simulink model "mpc_model_dual_module_allfreq"  (R2019a)
settings: Solver=FixedStepAuto  StartTime=0.0  StopTime=Tfinal  RelTol=1e-3
values from neighbouring files (symbols this model uses):
  A = [-0.0285 -0.0014; -0.0371 -0.1476]    [model.m]
  DCLINK_Cap = 1000e-12    (= 1e-09)    [mpc_model_parameters.m]    (also in mpc_model_parameters_dual_module.m = 0.001)
  FluxPM = MeanInducedVoltagePeak/(2*pi*100)    [mpc_model_parameters.m]    (also in mpc_model_parameters_dual_module.m)
  Inertia = 1e-2    (= 0.01)    [mpc_model_parameters.m]    (also in mpc_model_parameters_dual_module.m)
  iqrated = Trated/(1.5*PolePairs*FluxPM)    [mpc_model_parameters.m]    (also in mpc_model_parameters_dual_module.m)
  Ki = 8    [mpc_model_parameters_dual_module.m]
  Kp = 0.8    [mpc_model_parameters_dual_module.m]
  Ls = 3.5e-3    (= 0.0035)    [MPC_id_iq.m]    (also in mpc_model_parameters.m = 0.00351; mpc_model_parameters_dual_module.m = 0.00343)
  M1_FaultTime = 0.25    [mpc_model_parameters_dual_module.m]
  M2_FaultTime = 20    [mpc_model_parameters_dual_module.m]
  MeanLd = (1/12)*(Module1Phase_A_Ld+Module1Phase_B_Ld+Module1Phase_C_Ld+     Module2Phase_A_Ld+Module2Phase_B_Ld+Module2Phase_C_Ld+     Module3Phase_A_Ld+Module3Phase_B_Ld+Module3Phase_C_Ld+     Module4Phase_A_Ld+Module4Phase_B_Ld+Module4Phase_C_Ld)    [mpc_model_parameters.m]    (also in mpc_model_parameters_dual_module.m)
  MeanLq = (1/12)*(Module1Phase_A_Lq+Module1Phase_B_Lq+Module1Phase_C_Lq+     Module2Phase_A_Lq+Module2Phase_B_Lq+Module2Phase_C_Lq+     Module3Phase_A_Lq+Module3Phase_B_Lq+Module3Phase_C_Lq+     Module4Phase_A_Lq+Module4Phase_B_Lq+Module4Phase_C_Lq)    [mpc_model_parameters.m]    (also in mpc_model_parameters_dual_module.m)
  PI_Frequency = 5000    [mpc_model_parameters_dual_module.m]
  PI_Sat = iqrated*2    [mpc_model_parameters_dual_module.m]
  PI_Ts = 1/PI_Frequency    (= 0.0002)    [mpc_model_parameters_dual_module.m]
  PolePairs = 10    [mpc_model_parameters.m]    (also in mpc_model_parameters_dual_module.m)
  RefModeSelection = 1    [mpc_model_parameters_dual_module.m]
  Rin = 1e-3    (= 0.001)    [mpc_model_parameters.m]    (also in mpc_model_parameters_dual_module.m)
  Rs = 0.531    [Loss_Distribution.m]    (also in MPC_id_iq.m; mpc_model_parameters.m = 0.321; mpc_model_parameters_dual_module.m = 0.539)
  Sampling_time = 1e-6    (= 1e-06)    [mpc_model_parameters.m]    (also in mpc_model_parameters_dual_module.m)
  SpeedRef1 = 50    [mpc_model_parameters.m]    (also in mpc_model_parameters_dual_module.m = 35)
  SpeedRef2 = 100    [mpc_model_parameters.m]    (also in mpc_model_parameters_dual_module.m = 35)
  SpeedRefUpdateTime = 0.25    [mpc_model_parameters.m]    (also in mpc_model_parameters_dual_module.m = 1.75)
  Tload1 = 5    [mpc_model_parameters.m]    (also in mpc_model_parameters_dual_module.m = 30)
  Tload2 = 10    [mpc_model_parameters.m]    (also in mpc_model_parameters_dual_module.m = 63.6619772368)
  TloadUpdateTime = 0.5    [mpc_model_parameters.m]    (also in mpc_model_parameters_dual_module.m)
  Vdc = 50    [mpc_model_parameters.m]    (also in mpc_model_parameters_dual_module.m = 40)
  Vin = Vdc + Rin*(Pout/Vdc)    (= 50.04)    [mpc_model_parameters.m]    (also in mpc_model_parameters_dual_module.m = 40.05)
  ViscousFriction = 1e-3    (= 0.001)    [mpc_model_parameters.m]    (also in mpc_model_parameters_dual_module.m)
undefined symbols (not defined in the file or in its folder): DiscIntNeverNeededParam
libraries: powerlib x27, dspsigops x21, dspswit3 x19, powerlib_meascontrol x10, fl_lib x5, simulink x4, nesl_utility x3, sdl_lib x1
(part 3 of 3)

== matlab function mpc_model_dual_module_allfreq/MATLAB Function1 ==
  data: pulse input; inputwave input; outputwave output
function outputwave  = fcn(pulse, inputwave)

persistent state

if isempty(state)
state = 0;
end

if(pulse==1)
    state = state +1;
end

if(mod(state,2)==1)
    outputwave = inputwave;
    return;
end
if(mod(state,2)==0)
    outputwave = 1-inputwave;
    return;
end

outputwave = 5;

== matlab function mpc_model_dual_module_allfreq/MATLAB Function2 ==
  data: pulse input; inputwave input; outputwave output
function outputwave  = fcn(pulse, inputwave)

persistent state

if isempty(state)
state = 0;
end

if(pulse==1)
    state = state +1;
end

if(mod(state,2)==1)
    outputwave = inputwave;
    return;
end
if(mod(state,2)==0)
    outputwave = 1-inputwave;
    return;
end

outputwave = 5;

== matlab function mpc_model_dual_module_allfreq/module 1 abc to dq1 ==
  data: ids output; iqs output; ias input; ibs input; ics input; ref_frame_position input; i0 output
function [ids,iqs,i0 ]  = fcn(ias,ibs,ics,ref_frame_position)





ids = 2/3*(ias*sin(ref_frame_position)+ibs*sin(ref_frame_position-2*pi/3)+ics*sin(ref_frame_position+2*pi/3));
iqs =  2/3*(ias*cos(ref_frame_position)+ibs*cos(ref_frame_position-2*pi/3)+ics*cos(ref_frame_position+2*pi/3));
i0 = 2/3*1/2*(ias+ibs+ics);
% iqs = (vqs-fluxlinkage_qs_derivative-ref_frame_velocity*fluxlinkage_ds)/rs;
% ids = (vds-fluxlinkage_ds_derivative+ref_frame_velocity*fluxlinkage_qs)/rs;

== matlab function mpc_model_dual_module_allfreq/MATLAB Function4 ==
  data: M1_ia input; M1_loss output; M1_ib input; M1_ic input; M2_ia input; M2_ib input; M2_ic input; M2_loss output; Total_loss output; Rs input
function [M1_loss,M2_loss,Total_loss] = fcn(M1_ia, M1_ib, M1_ic, M2_ia, M2_ib, M2_ic, Rs)



M1_loss = Rs*(M1_ia^2+M1_ib^2+M1_ic^2);
M2_loss = Rs*(M2_ia^2+M2_ib^2+M2_ic^2);
Total_loss = M1_loss+M2_loss;

== matlab function mpc_model_dual_module_allfreq/MATLAB Function5 ==
  data: M1_ids input; M1_magnetic_loss output; M1_iqs input; M2_ids input; M2_iqs input; FluxPM input; Ls input; ElectricalSpeed input; M2_magnetic_loss output; Total_loss output
function [M1_magnetic_loss,M2_magnetic_loss,Total_loss] = fcn(M1_ids,M1_iqs,M2_ids,M2_iqs,FluxPM,Ls,ElectricalSpeed)

cfe = 1.55;
lambda = 1.55;
M1_d_axis_flux = Ls*M1_ids+FluxPM;
M1_q_axis_flux = Ls*M1_iqs;
M2_d_axis_flux = Ls*M2_ids+FluxPM;
M2_q_axis_flux = Ls*M2_iqs;

M1_magnetic_loss = cfe*power(abs(ElectricalSpeed),lambda)*(M1_d_axis_flux^2+M1_q_axis_flux^2);
M2_magnetic_loss = cfe*power(abs(ElectricalSpeed),lambda)*(M2_d_axis_flux^2+M2_q_axis_flux^2);

% M1_loss = Rs*(M1_ia^2+M1_ib^2+M1_ic^2);
% M2_loss = Rs*(M2_ia^2+M2_ib^2+M2_ic^2);
Total_loss = M1_magnetic_loss+M2_magnetic_loss;

== matlab function mpc_model_dual_module_allfreq/MATLAB Function6 ==
  data: pulse input; inputwave input; outputwave output
function outputwave  = fcn(pulse, inputwave)

persistent state

if isempty(state)
state = 0;
end

if(pulse==1)
    state = state +1;
end

if(mod(state,2)==1)
    outputwave = inputwave;
    return;
end
if(mod(state,2)==0)
    outputwave = 1-inputwave;
    return;
end

outputwave = 5;

== matlab function mpc_model_dual_module_allfreq/MATLAB Function7 ==
  data: M1_Iq_opt_cost input; M1_iqref output; M1_Id_opt_cost input; M2_Iq_opt_cost input; M2_Id_opt_cost input; M1_Iq_opt_proportional input; M1_Id_opt_proportional input; M2_Iq_opt_proportional input; M2_Id_opt_proportional input; M1_Iq_opt_equal input; M1_Id_opt_equal input; M2_Iq_opt_equal input; M2_Id_opt_equal input; M1_idref output; M2_iqref output; M2_idref output; selection input
function [M1_iqref, M1_idref, M2_iqref, M2_idref] = fcn(M1_Iq_opt_cost,M1_Id_opt_cost,M2_Iq_opt_cost,M2_Id_opt_cost...
    ,M1_Iq_opt_proportional,M1_Id_opt_proportional,M2_Iq_opt_proportional,M2_Id_opt_proportional,...
    M1_Iq_opt_equal,M1_Id_opt_equal,M2_Iq_opt_equal,M2_Id_opt_equal,selection)


if(selection==1)
    M1_iqref = M1_Iq_opt_cost;
    M1_idref = M1_Id_opt_cost;
    M2_iqref = M2_Iq_opt_cost;
    M2_idref = M2_Id_opt_cost;
    return
end


if(selection==2)
    M1_iqref = M1_Iq_opt_proportional;
    M1_idref = M1_Id_opt_proportional;
    M2_iqref = M2_Iq_opt_proportional;
    M2_idref = M2_Id_opt_proportional;
    return
end



if(selection==3)
    M1_iqref = M1_Iq_opt_equal;
    M1_idref = M1_Id_opt_equal;
    M2_iqref = M2_Iq_opt_equal;
    M2_idref = M2_Id_opt_equal;
    return
end



    M1_iqref = M1_Iq_opt_equal;
    M1_idref = M1_Id_opt_equal;
    M2_iqref = M2_Iq_opt_equal;
    M2_idref = M2_Id_opt_equal;

== matlab function mpc_model_dual_module_allfreq/MATLAB Function8 ==
  data: interrupt1 input; phase output; interrupt2 input; time1 input; time2 input; counter_prev input; counter output; phase_prev input
function [phase, counter ] = fcn(interrupt1, interrupt2,time1, time2,counter_prev,phase_prev)

counter_temp = counter_prev;
if(interrupt1 == 1)
    counter_temp = counter_temp +1;   
end

if(interrupt2 == 1)
    counter_temp = counter_temp +1;  
end

counter = counter_temp;

if(mod(counter,2)==1)
    phase = time1-time2;
else
    phase = phase_prev;
end

== matlab function mpc_model_dual_module_allfreq/MATLAB Function10 ==
  data: pulse input; inputwave input; outputwave output
function outputwave  = fcn(pulse, inputwave)

persistent state

if isempty(state)
state = 0;
end

if(pulse==1)
    state = state +1;
end

if(mod(state,2)==1)
    outputwave = inputwave;
    return;
end
if(mod(state,2)==0)
    outputwave = 1-inputwave;
    return;
end

outputwave = 5;

== matlab function mpc_model_dual_module_allfreq/MATLAB Function9 ==
  data: InterruptSignal input; Ref input; Measured input; Ki input; Output output; Kp input; Ts input; Sat input; Error output; ErrorPrev input; OutputPrev input
function [Output,Error] = fcn(InterruptSignal,Ref,Measured,Ki,Kp,Ts,Sat, ErrorPrev,OutputPrev)
Error=0;
Output = 0;

if(InterruptSignal ==1)
    Error = Ref-Measured;
    
    Output = OutputPrev + Kp*(Error-ErrorPrev)+Ts/2*Ki*((Error+ErrorPrev));
    %  iqref = iqref_prev + Kp*(Speed_Error-Speed_Error_prev)+Ts_PI/2*Ki*((Speed_Error+Speed_Error_prev));
    if(abs(Output)>(Sat))
        if(Output>0)
            Output = Sat;
        else
            Output = -(Sat);
        end
    end
else
    Output=OutputPrev;
    Error = ErrorPrev;
end

== matlab function mpc_model_dual_module_allfreq/module 2 abc to dq1 ==
  data: ids output; iqs output; ias input; ibs input; ics input; ref_frame_position input; i0 output
function [ids,iqs,i0 ]  = fcn(ias,ibs,ics,ref_frame_position)





ids = 2/3*(ias*sin(ref_frame_position)+ibs*sin(ref_frame_position-2*pi/3)+ics*sin(ref_frame_position+2*pi/3));
iqs =  2/3*(ias*cos(ref_frame_position)+ibs*cos(ref_frame_position-2*pi/3)+ics*cos(ref_frame_position+2*pi/3));
i0 = 2/3*1/2*(ias+ibs+ics);
% iqs = (vqs-fluxlinkage_qs_derivative-ref_frame_velocity*fluxlinkage_ds)/rs;
% ids = (vds-fluxlinkage_ds_derivative+ref_frame_velocity*fluxlinkage_qs)/rs;

== matlab function mpc_model_dual_module_allfreq/MATLAB Function12 ==
  data: M1_id input; M1_copper_loss output; M1_iq input; M2_id input; M2_iq input; M2_copper_loss output
function [M1_copper_loss, M2_copper_loss ] = fcn(M1_id, M1_iq, M2_id, M2_iq)

Rs = 0.539;

M1_copper_loss = 1.5*Rs*(M1_id^2+M1_iq^2);

M2_copper_loss = 1.5*Rs*(M2_id^2+M2_iq^2);

== matlab function mpc_model_dual_module_allfreq/MATLAB Function13 ==
  data: Switch_Current input; fsw input; ConductionLoss output; SwitchingLoss output
function  [ConductionLoss, SwitchingLoss] = fcn(Switch_Current,fsw)

Rds_on = 2e-3;
GateCurrent = 1;

Qgs2 = 6.3e-9;
Qgd = 6.7e-9;

ConductionLoss = 6*Rds_on*Switch_Current^2;
SwitchingLoss = 6*40*abs(Switch_Current)*fsw*(Qgs2+Qgd)/GateCurrent;
% y = u;

== matlab function mpc_model_dual_module_allfreq/MATLAB Function14 ==
  data: Switch_Current input; fsw input; ConductionLoss output; SwitchingLoss output
function  [ConductionLoss, SwitchingLoss] = fcn(Switch_Current,fsw)

Rds_on = 2e-3;
GateCurrent = 1;

Qgs2 = 6.3e-9;
Qgd = 6.7e-9;

ConductionLoss = 6*Rds_on*Switch_Current^2;
SwitchingLoss = 6*40*abs(Switch_Current)*fsw*(Qgs2+Qgd)/GateCurrent;
% y = u;
